simulink model "obstactleDetection"  (R2020a)
settings: Solver=FixedStepDiscrete  StartTime=0.0  StopTime=50.0  FixedStep=0.01  RelTol=1e-3
undefined symbols (not defined in the file or in its folder): motorIp, motorSp
libraries: mobileRoboticsTrainingLib x5
settings Model: Creator=Navyasree  LastModifiedBy=Navyasree

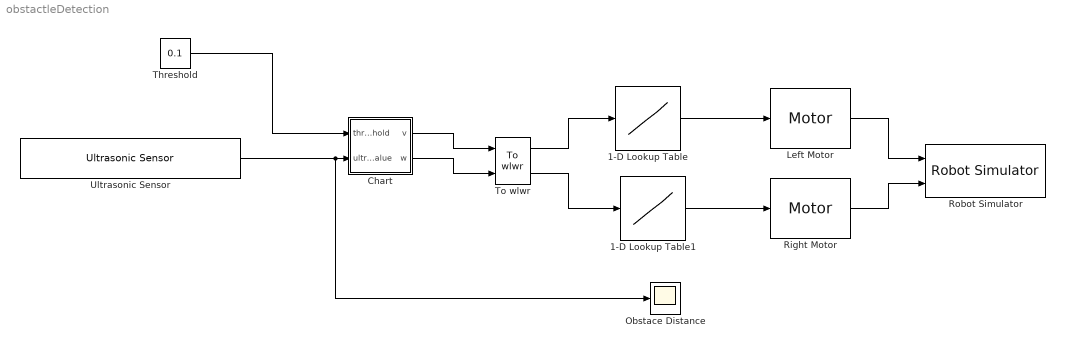
== system obstactleDetection ==
  1-D Lookup Table : Lookup_n-D  NumberOfTableDimensions=1  BreakpointsForDimension1=motorSp  Table=motorIp  InternalRulePriority=Speed  RndMeth=Simplest  InputSameDT=on
  1-D Lookup Table1 : Lookup_n-D  NumberOfTableDimensions=1  BreakpointsForDimension1=motorSp  Table=motorIp  InternalRulePriority=Speed  RndMeth=Simplest  InputSameDT=on
  Chart : Stateflow chart  TreatAsAtomicUnit=on
  Left Motor : mobileRoboticsTrainingLib/Motor  motorPlant=wheelMotorModel  sensorType=Speed
      settings: SourceProductName=Mobile Robotics Training Library
  Obstace Distance : Scope
  Right Motor : mobileRoboticsTrainingLib/Motor  motorPlant=wheelMotorModel  sensorType=Speed
      settings: SourceProductName=Mobile Robotics Training Library
  Robot Simulator : mobileRoboticsTrainingLib/Robot Simulator  Priority=99  mapVar=mapForSim  startX=2.6244  startY=0.9033  startTheta=90  axleLength=axleLength  wheelR=wheelR
  Threshold : Constant  Value=0.1
  To wlwr : mobileRoboticsTrainingLib/To wlwr  axleLength=0.1  wheelR=0.05
  Ultrasonic Sensor : mobileRoboticsTrainingLib/Ultrasonic Sensor  mapVar=mapForSim  maxSenRange=2  minSenRange=0.02  senRes=0.01  sensOff=[0 0]
      settings: SourceProductName=Mobile Robotics Training Library
  wires:
  To wlwr/1 -> 1-D Lookup Table/1
  1-D Lookup Table/1 -> Left Motor/1
  Left Motor/1 -> Robot Simulator/1
  Chart/1(v) -> To wlwr/1
  1-D Lookup Table1/1 -> Right Motor/1
  To wlwr/2 -> 1-D Lookup Table1/1
  Right Motor/1 -> Robot Simulator/2
  Ultrasonic Sensor/1 -> Obstace Distance/1, Chart/2(ultrasonicValue)
  Threshold/1 -> Chart/1(threshold)
  Chart/2(w) -> To wlwr/2

== stateflow chart obstactleDetection/Chart ==
  state GoForward
    entry: v=0.02
    w=0
  state Stop
    entry: v=0
    w=-1
  (default) -> GoForward
  GoForward -> Stop : [ultrasonicValue <= threshold]
  Stop -> GoForward : [ultrasonicValue > threshold]
  data: threshold input; ultrasonicValue input; v output; w output
